simulink model "labb4_3"  (R2019a)
settings: Solver=FixedStepAuto  StartTime=0.0  StopTime=0.2  FixedStep=0.01  RelTol=1e-3
settings Model: Creator=andfri18  LastModifiedBy=andfri18

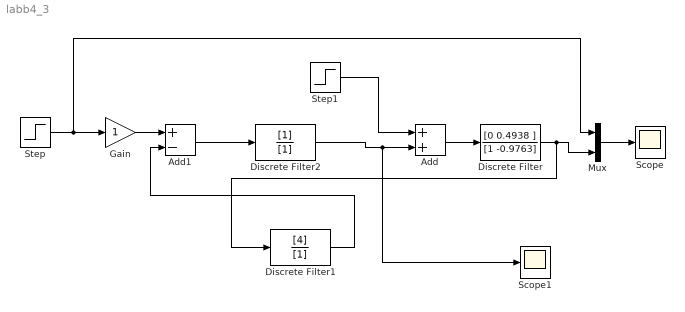
== system labb4_3 ==
  Add : Sum
  Add1 : Sum  Inputs=+-
  Discrete Filter : DiscreteFilter  Numerator=[0 0.4938 ]  Denominator=[1 -0.9763]
  Discrete Filter1 : DiscreteFilter  Numerator=[4]  Denominator=[1]
  Discrete Filter2 : DiscreteFilter  Denominator=[1]
  Gain : Gain
  Mux : Mux  Inputs=2
  Scope : Scope
  Scope1 : Scope
  Step : Step  Time=0.1
  Step1 : Step  Time=0  After=0  SampleTime=0
  wires:
  Mux/1 -> Scope/1
  Step1/1 -> Add/1
  Gain/1 -> Add1/1
  Step/1 -> Mux/1, Gain/1
  Add/1 -> Discrete Filter/1
  Discrete Filter/1 -> Discrete Filter1/1, Mux/2
  Discrete Filter1/1 -> Add1/2
  Add1/1 -> Discrete Filter2/1
  Discrete Filter2/1 -> Scope1/1, Add/2
